simulink model "robot_segway"  (R2023b)
settings: Solver=ode15s  StartTime=0.0  StopTime=tiempo_final  MaxStep=1e-3  RelTol=1e-5  AbsTol=1e-7
values from neighbouring files (symbols this model uses):
  Ts = se.Ts    [robot_controlador.m]    (also in simular_ode.m = P.sens.Ts; simular_slx.m = P.sens.Ts)
undefined symbols (not defined in the file or in its folder): estados_iniciales, medidas_iniciales, retardo_muestras, semilla
settings Model: Creator=calde  LastModifiedBy=calde

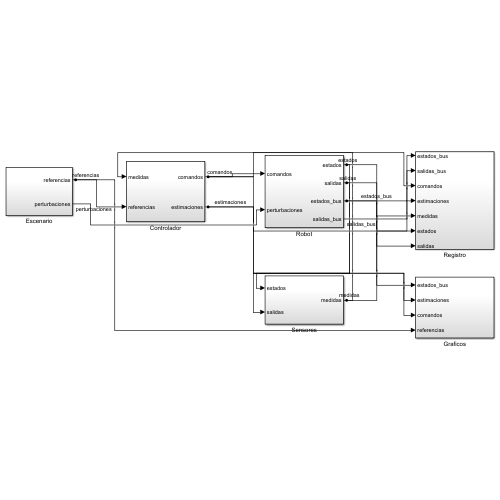
[thumbnail: Simulink's stored preview of the top-level diagram]
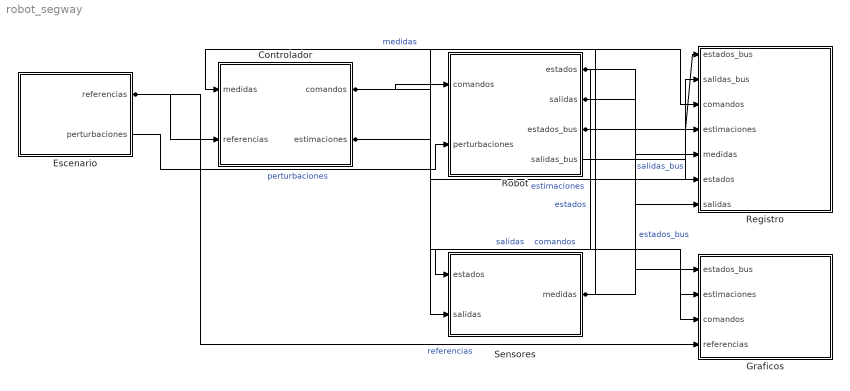
== system robot_segway ==
  Controlador : Subsystem
  Escenario : Subsystem
  Graficos : Subsystem
  Registro : Subsystem
  Robot : Subsystem
  Sensores : Subsystem
  wires:
  Escenario/1(referencias) -> Controlador/2(referencias), Graficos/4(referencias)  "referencias"
  Escenario/2(perturbaciones) -> Robot/2(perturbaciones)  "perturbaciones"
  Controlador/1(comandos) -> Robot/1(comandos), Registro/3(comandos), Graficos/3(comandos)  "comandos"
  Robot/1(estados) -> Sensores/1(estados), Registro/6(estados)  "estados"
  Robot/2(salidas) -> Sensores/2(salidas), Registro/7(salidas)  "salidas"
  Sensores/1(medidas) -> Controlador/1(medidas), Registro/5(medidas)  "medidas"
  Robot/3(estados_bus) -> Registro/1(estados_bus), Graficos/1(estados_bus)  "estados_bus"
  Robot/4(salidas_bus) -> Registro/2(salidas_bus)  "salidas_bus"
  Controlador/2(estimaciones) -> Registro/4(estimaciones), Graficos/2(estimaciones)  "estimaciones"

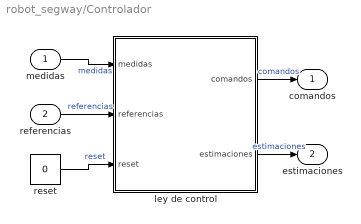
== system robot_segway/Controlador ==
  medidas : Inport
  referencias : Inport  Port=2
  ley de control : MATLAB Function  TreatAsAtomicUnit=on
  reset : Constant  Value=0  SampleTime=Ts
  comandos : Outport
  estimaciones : Outport  Port=2
  wires:
  referencias/1 -> ley de control/2(referencias)  "referencias"
  medidas/1 -> ley de control/1(medidas)  "medidas"
  reset/1 -> ley de control/3(reset)  "reset"
  ley de control/1(comandos) -> comandos/1  "comandos"
  ley de control/2(estimaciones) -> estimaciones/1  "estimaciones"

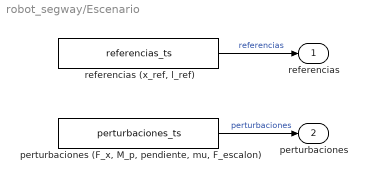
== system robot_segway/Escenario ==
  "perturbaciones (F_x, M_p, pendiente, mu, F_escalon)" : FromWorkspace  VariableName=perturbaciones_ts  Interpolate=off  OutputAfterFinalValue=Holding final value
  "referencias (x_ref, l_ref)" : FromWorkspace  VariableName=referencias_ts  SampleTime=Ts  Interpolate=off  OutputAfterFinalValue=Holding final value
  referencias : Outport
  perturbaciones : Outport  Port=2
  wires:
  "referencias (x_ref, l_ref)"/1 -> referencias/1  "referencias"
  "perturbaciones (F_x, M_p, pendiente, mu, F_escalon)"/1 -> perturbaciones/1  "perturbaciones"

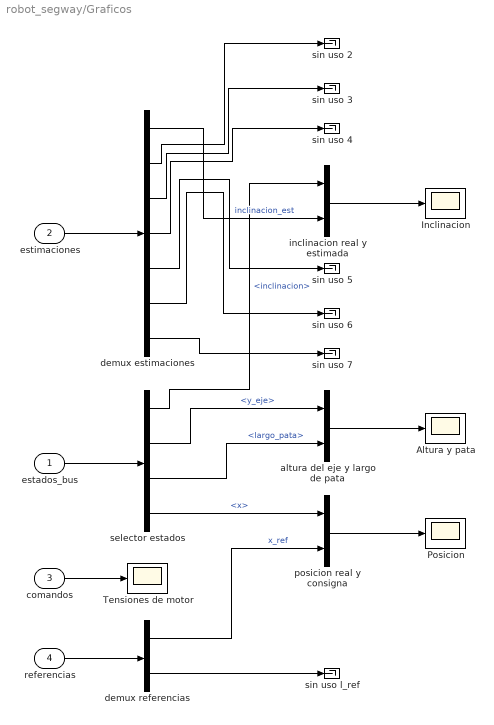
== system robot_segway/Graficos ==
  estados_bus : Inport
  estimaciones : Inport  Port=2
  comandos : Inport  Port=3
  referencias : Inport  Port=4
  Altura y pata : Scope
  Inclinacion : Scope
  Posicion : Scope
  Tensiones de motor : Scope
  altura del eje y largo de pata : Mux  Inputs=2
  demux estimaciones : Demux  Outputs=7
  demux referencias : Demux  Outputs=2
  inclinacion real y estimada : Mux  Inputs=2
  posicion real y consigna : Mux  Inputs=2
  selector estados : BusSelector  OutputSignals=inclinacion,y_eje,largo_pata,x
  sin uso {2..7} (6 alike) : Terminator
  sin uso l_ref : Terminator
  wires:
  demux estimaciones/1 -> inclinacion real y estimada/2  "inclinacion_est"
  estimaciones/1 -> demux estimaciones/1
  estados_bus/1 -> selector estados/1
  demux estimaciones/4 -> sin uso 4/1
  altura del eje y largo de pata/1 -> Altura y pata/1
  comandos/1 -> Tensiones de motor/1
  referencias/1 -> demux referencias/1
  demux estimaciones/2 -> sin uso 2/1
  demux estimaciones/3 -> sin uso 3/1
  demux estimaciones/5 -> sin uso 5/1
  demux estimaciones/6 -> sin uso 6/1
  demux estimaciones/7 -> sin uso 7/1
  selector estados/1 -> inclinacion real y estimada/1  "<inclinacion>"
  selector estados/2 -> altura del eje y largo de pata/1  "<y_eje>"
  selector estados/3 -> altura del eje y largo de pata/2  "<largo_pata>"
  selector estados/4 -> posicion real y consigna/1  "<x>"
  demux referencias/1 -> posicion real y consigna/2  "x_ref"
  demux referencias/2 -> sin uso l_ref/1
  inclinacion real y estimada/1 -> Inclinacion/1
  posicion real y consigna/1 -> Posicion/1

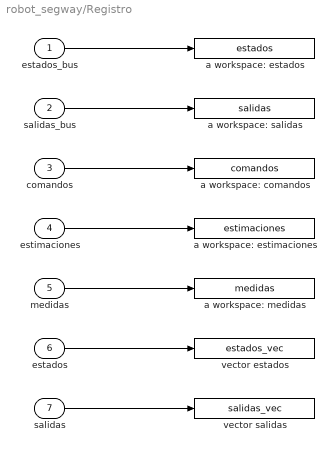
== system robot_segway/Registro ==
  estados_bus : Inport
  salidas_bus : Inport  Port=2
  comandos : Inport  Port=3
  estimaciones : Inport  Port=4
  medidas : Inport  Port=5
  estados : Inport  Port=6
  salidas : Inport  Port=7
  a workspace: comandos : ToWorkspace  VariableName=comandos  SaveFormat=Timeseries  SampleTime=-1
  a workspace: estados : ToWorkspace  VariableName=estados  SaveFormat=Timeseries  SampleTime=-1
  a workspace: estimaciones : ToWorkspace  VariableName=estimaciones  SaveFormat=Timeseries  SampleTime=-1
  a workspace: medidas : ToWorkspace  VariableName=medidas  SaveFormat=Timeseries  SampleTime=-1
  a workspace: salidas : ToWorkspace  VariableName=salidas  SaveFormat=Timeseries  SampleTime=-1
  vector estados : ToWorkspace  VariableName=estados_vec  SaveFormat=Structure With Time  SampleTime=-1
  vector salidas : ToWorkspace  VariableName=salidas_vec  SaveFormat=Structure With Time  SampleTime=-1
  wires:
  estados_bus/1 -> a workspace: estados/1
  salidas_bus/1 -> a workspace: salidas/1
  comandos/1 -> a workspace: comandos/1
  estimaciones/1 -> a workspace: estimaciones/1
  medidas/1 -> a workspace: medidas/1
  estados/1 -> vector estados/1
  salidas/1 -> vector salidas/1

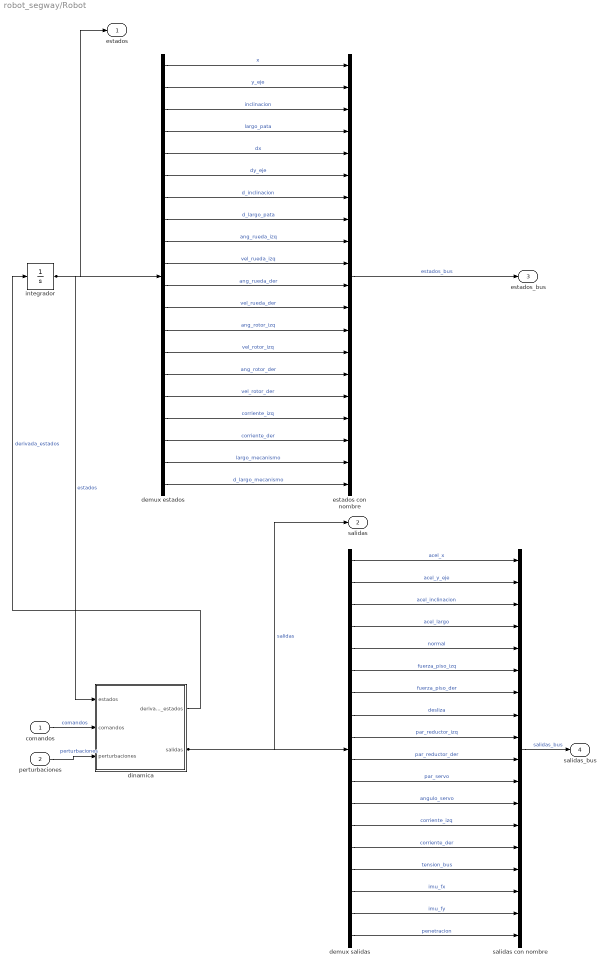
== system robot_segway/Robot ==
  comandos : Inport
  perturbaciones : Inport  Port=2
  demux estados : Demux  Outputs=20
  demux salidas : Demux  Outputs=18
  dinamica : MATLAB Function  TreatAsAtomicUnit=on
  estados con nombre : BusCreator  Inputs=20
  integrador : Integrator  InitialCondition=estados_iniciales
  salidas con nombre : BusCreator  Inputs=18
  estados : Outport
  salidas : Outport  Port=2
  estados_bus : Outport  Port=3
  salidas_bus : Outport  Port=4
  wires:
  integrador/1 -> estados/1, demux estados/1, dinamica/1(estados)  "estados"
  demux estados/5 -> estados con nombre/5  "dx"
  demux salidas/10 -> salidas con nombre/10  "par_reductor_der"
  demux estados/3 -> estados con nombre/3  "inclinacion"
  demux estados/10 -> estados con nombre/10  "vel_rueda_izq"
  comandos/1 -> dinamica/2(comandos)  "comandos"
  demux estados/2 -> estados con nombre/2  "y_eje"
  demux salidas/6 -> salidas con nombre/6  "fuerza_piso_izq"
  perturbaciones/1 -> dinamica/3(perturbaciones)  "perturbaciones"
  demux salidas/8 -> salidas con nombre/8  "desliza"
  demux estados/4 -> estados con nombre/4  "largo_pata"
  demux estados/1 -> estados con nombre/1  "x"
  demux estados/6 -> estados con nombre/6  "dy_eje"
  demux estados/7 -> estados con nombre/7  "d_inclinacion"
  demux estados/8 -> estados con nombre/8  "d_largo_pata"
  demux estados/9 -> estados con nombre/9  "ang_rueda_izq"
  demux estados/11 -> estados con nombre/11  "ang_rueda_der"
  demux salidas/13 -> salidas con nombre/13  "corriente_izq"
  demux estados/12 -> estados con nombre/12  "vel_rueda_der"
  demux salidas/11 -> salidas con nombre/11  "par_servo"
  dinamica/1(derivada_estados) -> integrador/1  "derivada_estados"
  demux estados/13 -> estados con nombre/13  "ang_rotor_izq"
  demux salidas/7 -> salidas con nombre/7  "fuerza_piso_der"
  demux estados/14 -> estados con nombre/14  "vel_rotor_izq"
  demux estados/15 -> estados con nombre/15  "ang_rotor_der"
  demux estados/16 -> estados con nombre/16  "vel_rotor_der"
  demux estados/20 -> estados con nombre/20  "d_largo_mecanismo"
  demux estados/17 -> estados con nombre/17  "corriente_izq"
  demux estados/18 -> estados con nombre/18  "corriente_der"
  demux salidas/1 -> salidas con nombre/1  "acel_x"
  demux estados/19 -> estados con nombre/19  "largo_mecanismo"
  estados con nombre/1 -> estados_bus/1  "estados_bus"
  dinamica/2(salidas) -> salidas/1, demux salidas/1  "salidas"
  demux salidas/2 -> salidas con nombre/2  "acel_y_eje"
  demux salidas/3 -> salidas con nombre/3  "acel_inclinacion"
  demux salidas/4 -> salidas con nombre/4  "acel_largo"
  demux salidas/5 -> salidas con nombre/5  "normal"
  demux salidas/9 -> salidas con nombre/9  "par_reductor_izq"
  demux salidas/12 -> salidas con nombre/12  "angulo_servo"
  demux salidas/14 -> salidas con nombre/14  "corriente_der"
  demux salidas/15 -> salidas con nombre/15  "tension_bus"
  demux salidas/16 -> salidas con nombre/16  "imu_fx"
  demux salidas/17 -> salidas con nombre/17  "imu_fy"
  demux salidas/18 -> salidas con nombre/18  "penetracion"
  salidas con nombre/1 -> salidas_bus/1  "salidas_bus"

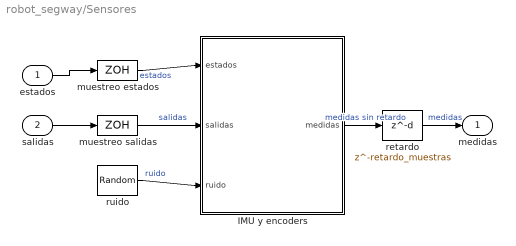
== system robot_segway/Sensores ==
  estados : Inport
  salidas : Inport  Port=2
  IMU y encoders : MATLAB Function  TreatAsAtomicUnit=on
  muestreo estados : ZeroOrderHold  SampleTime=Ts
  muestreo salidas : ZeroOrderHold  SampleTime=Ts
  retardo : Delay  DelayLength=retardo_muestras  InitialCondition=medidas_iniciales  SampleTime=Ts
  ruido : RandomNumber  Seed=semilla+[0 1 2]  SampleTime=Ts
  medidas : Outport
  wires:
  estados/1 -> muestreo estados/1
  salidas/1 -> muestreo salidas/1
  muestreo estados/1 -> IMU y encoders/1(estados)  "estados"
  muestreo salidas/1 -> IMU y encoders/2(salidas)  "salidas"
  ruido/1 -> IMU y encoders/3(ruido)  "ruido"
  retardo/1 -> medidas/1  "medidas"
  IMU y encoders/1(medidas) -> retardo/1  "medidas sin retardo"

== matlab function robot_segway/Robot/dinamica ==
  data: estados input; derivada_estados output; comandos input; perturbaciones input; salidas output; par parameter
function [derivada_estados, salidas] = fcn(estados, comandos, perturbaciones, par)
%#codegen
% estados (20): [x y_eje inclinacion largo_pata dx dy d_inclinacion d_largo ang/vel rueda izq-der ang/vel rotor izq-der corrientes largo_mecanismo d_largo_mecanismo]
% comandos = [tension_izq; tension_der; angulo_servo_ref]   perturbaciones = [F_x; M_p; pendiente; mu; F_escalon]
[derivada_estados, salidas] = robot_planta(estados, comandos, perturbaciones, par);

== matlab function robot_segway/Controlador/ley de control ==
  data: medidas input; comandos output; referencias input; reset input; estimaciones output; par parameter
function [comandos, estimaciones] = fcn(medidas, referencias, reset, par)
%#codegen
% medidas = [giroscopo; acel_x; acel_y; encoder_izq; encoder_der]   referencias = [x_ref; l_ref]
[comandos, estimaciones] = robot_controlador(medidas, referencias, par, reset);

== matlab function robot_segway/Sensores/IMU y encoders ==
  data: estados input; medidas output; salidas input; ruido input; par parameter
function medidas = fcn(estados, salidas, ruido, par)
%#codegen
% medidas = [giroscopo; acel_x; acel_y; encoder_izq; encoder_der]
medidas = robot_sensores(estados, salidas, ruido, par);
